simulink model "lmsdemo"  (Simulink 6.0)
settings: Solver=FixedStepDiscrete  StartTime=0  StopTime=inf  RelTol=1e-3  AbsTol=1e-6
libraries: dspsnks4 x2, simulink x2, dspsrcs4 x2, dspadpt3 x1, dsparch4 x1
Description:
  | LMS adaptive noise cancellation
settings Model: CovMetricSettings=d  Creator=don  LastModifiedBy=mkhan  ExtModeTrigMode=oneshot  ExtModeArmWhenConnect=off  ExtModeAutoUpdateStatusClock=off  ProdHWDeviceType=Specified
settings DataIOCC: LimitDataPoints=off  SaveOutput=off  SaveTime=off  SignalLoggingName=sigsOut
settings OptimizationCC: InlineInvariantSignals=off
settings DebuggingCC: CheckExecutionContextPreStartOutputMsg=on  CheckExecutionContextRuntimeOutputMsg=on  SolverPrmCheckMsg=none  IntegerOverflowMsg=none
settings HardwareCC: ProdBitPerShort=32  ProdBitPerInt=16  ProdHWDeviceType=Specified  TargetUnknown=on
settings SFSimCC: SFSimApplyToAllLibs=on  SFSimBuildMode=Incremental

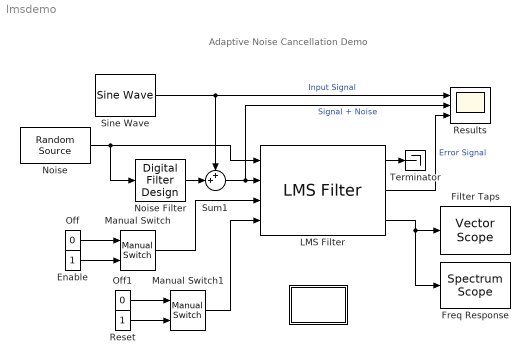
== system lmsdemo ==
  note: Adaptive Noise Cancellation Demo
  " " : Subsystem  PropExecContextAcrossSSBoundary=on
      mask Display: disp('Info')
  Enable : Constant  OutDataTypeMode=boolean
  Filter Taps : dspsnks4/Vector Scope  ScopeProperties=off  Domain=User-defined  HorizSpan=1  DisplayProperties=off  AxisGrid=on  Memory=off  FrameNumber=on  AxisLegend=off  AxisZoom=on  OpenScopeAtSimStart=on  OpenScopeImmediately=off  FigPos=[31 210 329 270]  AxisProperties=on  XUnits=Hertz  XRange=[0...Fs/2]  InheritXIncr=on  XIncr=1  XLabel=Samples  YUnits=dB  YLabel=Filter Coefficients  LineProperties=off  LineDisables=on  LineStyles=:  LineMarkers=.  LineColors=[0 0 1]
      settings: YMin=-0.2  YMax=0.6
  Freq Response : dspsnks4/Spectrum Scope  ScopeProperties=off  Domain=Frequency  HorizSpan=1  UseBuffer=off  BufferSize=128  Overlap=64  inpFftLenInherit=on  FFTlength=256  numAvg=2  DisplayProperties=off  AxisGrid=on  Memory=off  FrameNumber=on  AxisLegend=off  AxisZoom=on  OpenScopeAtSimStart=on  OpenScopeImmediately=off  FigPos=[372 208 378 270]  AxisProperties=on  XUnits=Hertz  XRange=[0...Fs/2]  InheritXIncr=on  XIncr=1  XLabel=Samples  YUnits=dB  YLabel=Magnitude, dB  LineProperties=off  LineDisables=on  LineStyles=-  LineColors=[0 0 1]
      settings: YMin=-60  YMax=0
  LMS Filter : dspadpt3/LMS Filter  DialogController=dspDDGCreate  DialogControllerArgs=DataTag0  Algo=Normalized LMS  L=32  stepflag=Dialog  mu=0.1  leakage=1.0  ic=0  Adapt=on  resetflag=Either edge  weights=on  secondCoeffMode=User-defined  secondCoeffWordLength=2  secondCoeffFracLength=15  accum2Mode=User-defined  accum2FracLength=20  prodOutput2Mode=User-defined  prodOutput2FracLength=20  prodOutput3Mode=User-defined  prodOutput3FracLength=20  prodOutput4Mode=User-defined  prodOutput4FracLength=20  quotientMode=User-defined  quotientFracLength=20  roundingMode=Floor  overflowMode=off  addnparflag=on
  Manual Switch : simulink/Signal Routing/Manual Switch  sw=0  action=0
  Manual Switch1 : simulink/Signal Routing/Manual Switch  sw=1  action=0
  Noise : dspsrcs4/Random Source  SrcType=Gaussian  NormMethod=Ziggurat  CltLength=12  Min=0  Max=1  Mean=0  Var=1  RepMode=Specify seed  rawSeed=[23341]  Inherit=off  SampMode=Discrete  SampTime=1  SampFrame=1  DataType=Double  OutComplex=Real
  Noise Filter : dsparch4/Digital Filter Design
  Off : Constant  Value=0  OutDataTypeMode=boolean
  Off1 : Constant  Value=0  OutDataTypeMode=boolean
  Reset : Constant  OutDataTypeMode=boolean
  Results : Scope  NumInputPorts=3
      settings: TimeRange=128  YMin=-2~-2~-2  YMax=2~2~2  DataFormat=Array
  Sine Wave : dspsrcs4/Sine Wave  Amplitude=1  Frequency=0.055  Phase=0  SampleMode=Discrete  OutComplex=Real  CompMethod=Trigonometric fcn  TableSize=Speed  SampleTime=1  SamplesPerFrame=1  dataType=double  wordLen=16  udDataType=sfix(16)  fracBitsMode=User-defined  numFracBits=14  ResetState=Restart at time zero
  Sum1 : Sum  Inputs=++|  SaturateOnIntegerOverflow=on  InputSameDT=on
  Terminator : Terminator
  wires:
  Sine Wave/1 -> Results/1, Sum1/1  "Input Signal"
  Noise Filter/1 -> Sum1/2
  Noise/1 -> LMS Filter/1, Noise Filter/1
  Sum1/1 -> Results/2, LMS Filter/2  "Signal + Noise"
  LMS Filter/2 -> Results/3  "Error Signal"
  LMS Filter/1 -> Terminator/1
  LMS Filter/3 -> Freq Response/1, Filter Taps/1
  Off/1 -> Manual Switch/1
  Enable/1 -> Manual Switch/2
  Off1/1 -> Manual Switch1/1
  Reset/1 -> Manual Switch1/2
  Manual Switch/1 -> LMS Filter/3
  Manual Switch1/1 -> LMS Filter/4

== system lmsdemo/  ==
  note: Adaptive Noise Cancellation using the Least
      | Mean Square Algorithm
      |
      | The LMS adaptive filter uses the reference signal (on
      | the "Input" port) and the desired signal (on the "Desired" port) to automatically
      |  match the filter response in the block labeled "Noise filter".
      |  As it converges to the correct filter, the filtered noise should
      |  be completely subtracted from the "Signal + Noise" signal and
      | the "Error Signal" should contain only the original signal.
      |
      | For details, see "Adaptive Filter Theory", 3rd Ed. by
      | S. Haykin, Prentice-Hall 1996.
